simulink library "simCryogenics_lib"  (R2016a)
settings: Solver=VariableStepAuto  StartTime=0.0  StopTime=10.0  RelTol=1e-3
undefined symbols (not defined in the file or in its folder): gcbh, simscape
(part 3 of 4)

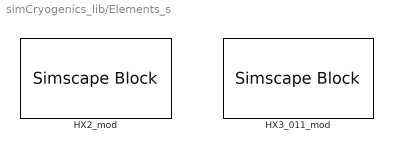
== system simCryogenics_lib/Elements_s ==
  HX2_mod : SimscapeBlock  DialogController=NetworkEngine.DynNeDlgSource  LoadFcn=simscape.compiler.sli.internal.callback('LoadFcn',gcbh);  SourceFile=simCryogenics.Elements_s.HeatEx2_mod  mask(HX2_mod){ComponentPath=simCryogenics.Elements_s.HeatEx2_mod, ComponentVariants=simCryogenics.Elements_s.HeatEx2_mod, ComponentVariantNames=HeatEx2_mod, ClassName=HeatEx2_mod, SchemaVersion=1, N=1, N_unit=1, N_conf=compiletime, Vh=2.3e-3, Vh_unit=m^3, Vh_conf=compiletime, Vc=2.3e-3, Vc_unit=m^3, Vc_conf=compiletime, M=13, M_unit=kg, M_conf=compiletime, Kh=0.6, Kh_unit=s*bar/kg, Kh_conf=compiletime, Kc=0.35, Kc_unit=s*bar/kg, Kc_conf=compiletime, Th0=10, Th0_unit=K, Th0_conf=compiletime, Ph0=16, Ph0_unit=bar, Ph0_conf=compiletime, Mh0=0.037, Mh0_unit=kg/s, Mh0_conf=compiletime, Tc0=4.5, Tc0_unit=K, Tc0_conf=compiletime, Pc0=1.1, Pc0_unit=bar, Pc0_conf=compiletime, Mc0=0.037, Mc0_unit=kg/s, Mc0_conf=compiletime, hhn=480, hhn_unit=J/s/K, hhn_conf=compiletime, hcn=480, hcn_unit=J/s/K, hcn_conf=compiletime, Mhn=1, Mhn_unit=kg/s, Mhn_conf=compiletime, Mcn=1, Mcn_unit=kg/s, Mcn_conf=compiletime, Thn=10, Thn_unit=K, Thn_conf=compiletime, Tcn=4.5, Tcn_unit=K, Tcn_conf=compiletime, Phn=16, Phn_unit=bar, Phn_conf=compiletime, Pcn=1.1, Pcn_unit=bar, Pcn_conf=compiletime, ex_mode=1, ex_mode_unit=1, ex_mode_conf=compiletime}
      mask prompts: N "Number of discrete elements"; Vh "First passage volume"; Vc "Sec. passage volume"; M "Heat exchanger mass"; Kh "First passage press. drop coeff."; Kc "Sec. passage press. drop coeff."; Th0 "Initial in1 temperature"; Ph0 "Initial in1 pressure"; Mh0 "Initial out1 flowrate"; Tc0 "Initial in2 temperature"; Pc0 "Initial out2 pressure"; Mc0 "Initial in2 flowrate"; hhn "Nominal exchange coefficient for hot pipe"; hcn "Nominal exchange coefficient for cold pipe"; Mhn "Nominal hot pipe flowrate"; Mcn "Nominal cold pipe flowrate"; Thn "Nominal hot pipe temperature"; Tcn "Nominal cold pipe temperature"; Phn "Nominal hot pipe pressure"; Pcn "Nominal cold pipe pressure"; ex_mode "Choice for h computation"
      mask help:
      | This component is a two branches cross-current heat Exchanger
      |
      | The following variables are imposed to others components: - in1 node : flow rate - out1 node : pressure and enthalpy - in2 node : enthalpy and flow rate - out2 node : pressure
      |
      | To ensure compilation, the heat Exchanger must be connected to components nodes that impose: - pressure and enthalpy on the in1 node - flowrate on the out1 node - flowrate and enthalpy on the in2 node - pressure on the out2 node
      |
      | Note : the initial temperature/flowrate/presure conditions should be equal to the actual value on the scheme (especially for heat exchangers connected to sources).
      |
      | All parameters must be positive
      mask init:
      | simscape.compiler.sli.internal.preinitmask(gcb);
      settings: CopyFcn=simscape.compiler.sli.internal.callback('CopyFcn',gcbh);  DeleteFcn=simscape.compiler.sli.internal.callback('DeleteFcn',gcbh);  ModelCloseFcn=simscape.compiler.sli.internal.callback('ModelCloseFcn',gcbh);  PreSaveFcn=simscape.compiler.sli.internal.callback('PreSaveFcn',gcbh);  PostSaveFcn=simscape.compiler.sli.internal.callback('PostSaveFcn',gcbh);  PreCopyFcn=simscape.compiler.sli.internal.callback('PreCopyFcn',gcbh);  PreDeleteFcn=simscape.compiler.sli.internal.callback('PreDeleteFcn',gcbh);
      mask Help: web(nesl_help(gcbh))
      mask TypeOptions N_conf: compiletime
      mask TypeOptions Vh_conf: compiletime
      mask TypeOptions Vc_conf: compiletime
      mask TypeOptions M_conf: compiletime
      mask TypeOptions Kh_conf: compiletime
      mask TypeOptions Kc_conf: compiletime
      mask TypeOptions Th0_conf: compiletime
      mask TypeOptions Ph0_conf: compiletime
      mask TypeOptions Mh0_conf: compiletime
      mask TypeOptions Tc0_conf: compiletime
      mask TypeOptions Pc0_conf: compiletime
      mask TypeOptions Mc0_conf: compiletime
      mask TypeOptions hhn_conf: compiletime
      mask TypeOptions hcn_conf: compiletime
      mask TypeOptions Mhn_conf: compiletime
      mask TypeOptions Mcn_conf: compiletime
      mask TypeOptions Thn_conf: compiletime
      mask TypeOptions Tcn_conf: compiletime
      mask TypeOptions Phn_conf: compiletime
      mask TypeOptions Pcn_conf: compiletime
      mask TypeOptions ex_mode_conf: compiletime | runtime
      mask Display:
      | disp('Simscape\n\n\n')
      | disp('\n\n\nHeatEx2_mod');
      | color('red');
      | port_label('RConn', 2,'out1');
      | port_label('RConn', 1,'in2');
      | port_label('LConn', 2,'in1');
      | port_label('LConn', 1,'out2');
  HX3_011_mod : SimscapeBlock  DialogController=NetworkEngine.DynNeDlgSource  LoadFcn=simscape.compiler.sli.internal.callback('LoadFcn',gcbh);  SourceFile=simCryogenics.Elements_s.HeatEx3_011_mod  mask(HX3_011_mod){ComponentPath=simCryogenics.Elements_s.HeatEx3_011_mod, ComponentVariants=simCryogenics.Elements_s.HeatEx3_011_mod, ComponentVariantNames=HeatEx3_011_mod, ClassName=HeatEx3_011_mod, SchemaVersion=1, N=8, N_unit=1, N_conf=compiletime, Vh=2.3e-3, Vh_unit=m^3, Vh_conf=compiletime, Vm=2.3e-3, Vm_unit=m^3, Vm_conf=compiletime, Vc=2.3e-3, Vc_unit=m^3, Vc_conf=compiletime, M=13, M_unit=kg, M_conf=compiletime, Kh=0, Kh_unit=s*bar/kg, Kh_conf=compiletime, Km=0, Km_unit=s*bar/kg, Km_conf=compiletime, Kc=0, Kc_unit=s*bar/kg, Kc_conf=compiletime, hn_h=400, hn_h_unit=W/K, hn_h_conf=compiletime, hn_m=400, hn_m_unit=W/K, hn_m_conf=compiletime, hn_c=400, hn_c_unit=W/K, hn_c_conf=compiletime, Th0=10, Th0_unit=K, Th0_conf=compiletime, Ph0=16, Ph0_unit=bar, Ph0_conf=compiletime, Mh0=0.037, Mh0_unit=kg/s, Mh0_conf=compiletime, Tm0=4.5, Tm0_unit=K, Tm0_conf=compiletime, Pm0=1.1, Pm0_unit=bar, Pm0_conf=compiletime, Mm0=0.037, Mm0_unit=kg/s, Mm0_conf=compiletime, Tc0=4.5, Tc0_unit=K, Tc0_conf=compiletime, Pc0=1.1, Pc0_unit=bar, Pc0_conf=compiletime, Mc0=0.037, Mc0_unit=kg/s, Mc0_conf=compiletime, Thn=10, Thn_unit=K, Thn_conf=compiletime, Phn=16, Phn_unit=bar, Phn_conf=compiletime, Mhn=0.037, Mhn_unit=kg/s, Mhn_conf=compiletime, Tmn=4.5, Tmn_unit=K, Tmn_conf=compiletime, Pmn=1.1, Pmn_unit=bar, Pmn_conf=compiletime, Mmn=0.037, Mmn_unit=kg/s, Mmn_conf=compiletime, Tcn=4.5, Tcn_unit=K, Tcn_conf=compiletime, Pcn=1.1, Pcn_unit=bar, Pcn_conf=compiletime, Mcn=0.037, Mcn_unit=kg/s, Mcn_conf=compiletime, ex_hp_bp=10, ex_hp_bp_unit=1, ex_hp_bp_conf=compiletime, ex_hp_mp=10, ex_hp_mp_unit=1, ex_hp_mp_conf=compiletime, ex_mp_bp=10, ex_mp_bp_unit=1, ex_mp_bp_conf=compiletime, ex_mode=1, ex_mode_unit=1, ex_mode_conf=compiletime, sensh=0, sensh_unit=1, sensh_conf=compiletime, sensm=1, sensm_unit=1, sensm_conf=compiletime, sensc=1, sensc_unit=1, sensc_conf=compiletime}
      mask prompts: N "Number of discrete elements"; Vh "First passage volume"; Vm "Second passage volume"; Vc "Third passage volume"; M "Heat exchanger mass"; Kh "First passage pressure drop"; Km "Second passage pressure drop"; Kc "Third passage pressure drop"; hn_h "Nominal ex. coef. for HP stream"; hn_m "Nominal ex. coef. for MP stream"; hn_c "Nominal ex. coef. for BP stream"; Th0 "Initial in1 temperature"; Ph0 "Initial in1 pressure"; Mh0 "Initial out1 flowrate"; Tm0 "Initial in2 temperature"; Pm0 "Initial out2 pressure"; Mm0 "Initial in2 flowrate"; Tc0 "Initial in3 temperature"; Pc0 "Initial out3 pressure"; Mc0 "Initial in3 flowrate"; Thn "Nominal in1 temperature"; Phn "Nominal in1 pressure"; Mhn "Nominal out1 flowrate"; Tmn "Nominal in2 temperature"; Pmn "Nominal out2 pressure"; Mmn "Nominal in2 flowrate"; Tcn "Nominal in3 temperature"; Pcn "Nominal out3 pressure"; Mcn "Nominal in3 flowrate"; ex_hp_bp "Number of interfaces between HP and BP streams"; ex_hp_mp "Number of interfaces between HP and MP streams"; ex_mp_bp "Number of interfaces between MP and BP streams"; ex_mode "Choice for h computation"; sensh "Sens hot flow"; sensm "Sens middle flow"; sensc "Sens cold flow"
      mask help:
      | This component is a three branches cross-current heat Exchanger
      |
      | The following variables are imposed to others components: - in1 node : pressure and enthalpy - out1 node :  flow rate - in2/3 node : enthalpy and flow rate - out2/3 node : pressure
      |
      | To ensure compilation, the heat Exchanger must be connected to components nodes that impose: - pressure and enthalpy on the in1 node - flowrate on the out1 node - flowrate and enthalpy on the in2/3 node - pressure on the out2/3 node
      |
      | Note : the initial temperature/flowrate/presure conditions should be equal to the actual value on the scheme (especially for heat exchangers connected to sources).
      |
      | All parameters must be positive
      mask init:
      | simscape.compiler.sli.internal.preinitmask(gcb);
      settings: CopyFcn=simscape.compiler.sli.internal.callback('CopyFcn',gcbh);  DeleteFcn=simscape.compiler.sli.internal.callback('DeleteFcn',gcbh);  ModelCloseFcn=simscape.compiler.sli.internal.callback('ModelCloseFcn',gcbh);  PreSaveFcn=simscape.compiler.sli.internal.callback('PreSaveFcn',gcbh);  PostSaveFcn=simscape.compiler.sli.internal.callback('PostSaveFcn',gcbh);  PreCopyFcn=simscape.compiler.sli.internal.callback('PreCopyFcn',gcbh);  PreDeleteFcn=simscape.compiler.sli.internal.callback('PreDeleteFcn',gcbh);
      mask Help: web(nesl_help(gcbh))
      mask TypeOptions N_conf: compiletime
      mask TypeOptions Vh_conf: compiletime
      mask TypeOptions Vm_conf: compiletime
      mask TypeOptions Vc_conf: compiletime
      mask TypeOptions M_conf: compiletime
      mask TypeOptions Kh_conf: compiletime
      mask TypeOptions Km_conf: compiletime
      mask TypeOptions Kc_conf: compiletime
      mask TypeOptions hn_h_conf: compiletime
      mask TypeOptions hn_m_conf: compiletime
      mask TypeOptions hn_c_conf: compiletime
      mask TypeOptions Th0_conf: compiletime
      mask TypeOptions Ph0_conf: compiletime
      mask TypeOptions Mh0_conf: compiletime
      mask TypeOptions Tm0_conf: compiletime
      mask TypeOptions Pm0_conf: compiletime
      mask TypeOptions Mm0_conf: compiletime
      mask TypeOptions Tc0_conf: compiletime
      mask TypeOptions Pc0_conf: compiletime
      mask TypeOptions Mc0_conf: compiletime
      mask TypeOptions Thn_conf: compiletime
      mask TypeOptions Phn_conf: compiletime
      mask TypeOptions Mhn_conf: compiletime
      mask TypeOptions Tmn_conf: compiletime
      mask TypeOptions Pmn_conf: compiletime
      mask TypeOptions Mmn_conf: compiletime
      mask TypeOptions Tcn_conf: compiletime
      mask TypeOptions Pcn_conf: compiletime
      mask TypeOptions Mcn_conf: compiletime
      mask TypeOptions ex_hp_bp_conf: compiletime
      mask TypeOptions ex_hp_mp_conf: compiletime
      mask TypeOptions ex_mp_bp_conf: compiletime
      mask TypeOptions ex_mode_conf: compiletime | runtime
      mask TypeOptions sensh_conf: compiletime
      mask TypeOptions sensm_conf: compiletime
      mask TypeOptions sensc_conf: compiletime
      mask Display:
      | disp('Simscape\n\n\n')
      | disp('\n\n\nHeatEx3_011_mod');
      | color('red');
      | port_label('LConn', 3,'in1');
      | port_label('LConn', 2,'out2');
      | port_label('LConn', 1,'out3');
      | port_label('RConn', 3,'out1');
      | port_label('RConn', 2,'in2');
      | port_label('RConn', 1,'in3');

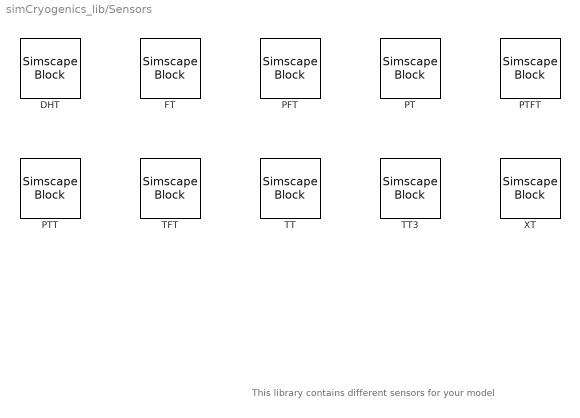
== system simCryogenics_lib/Sensors ==
  note: This library contains different sensors for your model
  DHT : SimscapeBlock  DialogController=NetworkEngine.DynNeDlgSource  LoadFcn=simscape.compiler.sli.internal.callback('LoadFcn',gcbh);  SourceFile=simCryogenics.Sensors.DHT  mask(DHT){ComponentPath=simCryogenics.Sensors.DHT, ComponentVariants=simCryogenics.Sensors.DHT, ComponentVariantNames=DHT, ClassName=DHT, SchemaVersion=1}
      mask init:
      | simscape.compiler.sli.internal.preinitmask(gcb);
      settings: CopyFcn=simscape.compiler.sli.internal.callback('CopyFcn',gcbh);  DeleteFcn=simscape.compiler.sli.internal.callback('DeleteFcn',gcbh);  ModelCloseFcn=simscape.compiler.sli.internal.callback('ModelCloseFcn',gcbh);  PreSaveFcn=simscape.compiler.sli.internal.callback('PreSaveFcn',gcbh);  PostSaveFcn=simscape.compiler.sli.internal.callback('PostSaveFcn',gcbh);  PreCopyFcn=simscape.compiler.sli.internal.callback('PreCopyFcn',gcbh);  PreDeleteFcn=simscape.compiler.sli.internal.callback('PreDeleteFcn',gcbh);
      mask Help: web(nesl_help(gcbh))
      mask Display:
      | color('red');
      | port_label('RConn', 1,'');
      | port_label('LConn', 2,'');
      | port_label('LConn', 1,'');
  FT : SimscapeBlock  DialogController=NetworkEngine.DynNeDlgSource  LoadFcn=simscape.compiler.sli.internal.callback('LoadFcn',gcbh);  SourceFile=simCryogenics.Sensors.FT  mask(FT){ComponentPath=simCryogenics.Sensors.FT, ComponentVariants=simCryogenics.Sensors.FT, ComponentVariantNames=FT, ClassName=FT, SchemaVersion=1}
      mask help: This component is a perfect flow sensor
      mask init:
      | simscape.compiler.sli.internal.preinitmask(gcb);
      settings: CopyFcn=simscape.compiler.sli.internal.callback('CopyFcn',gcbh);  DeleteFcn=simscape.compiler.sli.internal.callback('DeleteFcn',gcbh);  ModelCloseFcn=simscape.compiler.sli.internal.callback('ModelCloseFcn',gcbh);  PreSaveFcn=simscape.compiler.sli.internal.callback('PreSaveFcn',gcbh);  PostSaveFcn=simscape.compiler.sli.internal.callback('PostSaveFcn',gcbh);  PreCopyFcn=simscape.compiler.sli.internal.callback('PreCopyFcn',gcbh);  PreDeleteFcn=simscape.compiler.sli.internal.callback('PreDeleteFcn',gcbh);
      mask Help: web(nesl_help(gcbh))
      mask Display:
      | color('red');
      | port_label('RConn', 1,'');
      | port_label('LConn', 1,'');
  PFT : SimscapeBlock  DialogController=NetworkEngine.DynNeDlgSource  LoadFcn=simscape.compiler.sli.internal.callback('LoadFcn',gcbh);  SourceFile=simCryogenics.Sensors.PFT  mask(PFT){ComponentPath=simCryogenics.Sensors.PFT, ComponentVariants=simCryogenics.Sensors.PFT, ComponentVariantNames=PFT, ClassName=PFT, SchemaVersion=1}
      mask help: This component is a perfect pressure and temperature sensor
      mask init:
      | simscape.compiler.sli.internal.preinitmask(gcb);
      settings: CopyFcn=simscape.compiler.sli.internal.callback('CopyFcn',gcbh);  DeleteFcn=simscape.compiler.sli.internal.callback('DeleteFcn',gcbh);  ModelCloseFcn=simscape.compiler.sli.internal.callback('ModelCloseFcn',gcbh);  PreSaveFcn=simscape.compiler.sli.internal.callback('PreSaveFcn',gcbh);  PostSaveFcn=simscape.compiler.sli.internal.callback('PostSaveFcn',gcbh);  PreCopyFcn=simscape.compiler.sli.internal.callback('PreCopyFcn',gcbh);  PreDeleteFcn=simscape.compiler.sli.internal.callback('PreDeleteFcn',gcbh);
      mask Help: web(nesl_help(gcbh))
      mask Display:
      | color('red');
      | port_label('RConn', 2,'F');
      | port_label('RConn', 1,'P');
      | port_label('LConn', 1,'');
  PT : SimscapeBlock  DialogController=NetworkEngine.DynNeDlgSource  LoadFcn=simscape.compiler.sli.internal.callback('LoadFcn',gcbh);  SourceFile=simCryogenics.Sensors.PT  mask(PT){ComponentPath=simCryogenics.Sensors.PT, ComponentVariants=simCryogenics.Sensors.PT, ComponentVariantNames=PT, ClassName=PT, SchemaVersion=1}
      mask help: This component is a perfect pressure sensor
      mask init:
      | simscape.compiler.sli.internal.preinitmask(gcb);
      settings: CopyFcn=simscape.compiler.sli.internal.callback('CopyFcn',gcbh);  DeleteFcn=simscape.compiler.sli.internal.callback('DeleteFcn',gcbh);  ModelCloseFcn=simscape.compiler.sli.internal.callback('ModelCloseFcn',gcbh);  PreSaveFcn=simscape.compiler.sli.internal.callback('PreSaveFcn',gcbh);  PostSaveFcn=simscape.compiler.sli.internal.callback('PostSaveFcn',gcbh);  PreCopyFcn=simscape.compiler.sli.internal.callback('PreCopyFcn',gcbh);  PreDeleteFcn=simscape.compiler.sli.internal.callback('PreDeleteFcn',gcbh);
      mask Help: web(nesl_help(gcbh))
      mask Display:
      | color('red');
      | port_label('RConn', 1,'');
      | port_label('LConn', 1,'');
  PTFT : SimscapeBlock  DialogController=NetworkEngine.DynNeDlgSource  LoadFcn=simscape.compiler.sli.internal.callback('LoadFcn',gcbh);  SourceFile=simCryogenics.Sensors.PTFT  mask(PTFT){ComponentPath=simCryogenics.Sensors.PTFT, ComponentVariants=simCryogenics.Sensors.PTFT, ComponentVariantNames=PTFT, ClassName=PTFT, SchemaVersion=1}
      mask help: This component is a perfect pressure and temperature sensor
      mask init:
      | simscape.compiler.sli.internal.preinitmask(gcb);
      settings: CopyFcn=simscape.compiler.sli.internal.callback('CopyFcn',gcbh);  DeleteFcn=simscape.compiler.sli.internal.callback('DeleteFcn',gcbh);  ModelCloseFcn=simscape.compiler.sli.internal.callback('ModelCloseFcn',gcbh);  PreSaveFcn=simscape.compiler.sli.internal.callback('PreSaveFcn',gcbh);  PostSaveFcn=simscape.compiler.sli.internal.callback('PostSaveFcn',gcbh);  PreCopyFcn=simscape.compiler.sli.internal.callback('PreCopyFcn',gcbh);  PreDeleteFcn=simscape.compiler.sli.internal.callback('PreDeleteFcn',gcbh);
      mask Help: web(nesl_help(gcbh))
      mask Display:
      | color('red');
      | port_label('RConn', 3,'F');
      | port_label('RConn', 2,'T');
      | port_label('RConn', 1,'P');
      | port_label('LConn', 1,'');
  PTT : SimscapeBlock  DialogController=NetworkEngine.DynNeDlgSource  LoadFcn=simscape.compiler.sli.internal.callback('LoadFcn',gcbh);  SourceFile=simCryogenics.Sensors.PTT  mask(PTT){ComponentPath=simCryogenics.Sensors.PTT, ComponentVariants=simCryogenics.Sensors.PTT, ComponentVariantNames=PTT, ClassName=PTT, SchemaVersion=1}
      mask help: This component is a perfect pressure and temperature sensor
      mask init:
      | simscape.compiler.sli.internal.preinitmask(gcb);
      settings: CopyFcn=simscape.compiler.sli.internal.callback('CopyFcn',gcbh);  DeleteFcn=simscape.compiler.sli.internal.callback('DeleteFcn',gcbh);  ModelCloseFcn=simscape.compiler.sli.internal.callback('ModelCloseFcn',gcbh);  PreSaveFcn=simscape.compiler.sli.internal.callback('PreSaveFcn',gcbh);  PostSaveFcn=simscape.compiler.sli.internal.callback('PostSaveFcn',gcbh);  PreCopyFcn=simscape.compiler.sli.internal.callback('PreCopyFcn',gcbh);  PreDeleteFcn=simscape.compiler.sli.internal.callback('PreDeleteFcn',gcbh);
      mask Help: web(nesl_help(gcbh))
      mask Display:
      | color('red');
      | port_label('RConn', 2,'T');
      | port_label('RConn', 1,'P');
      | port_label('LConn', 1,'');
  TFT : SimscapeBlock  DialogController=NetworkEngine.DynNeDlgSource  LoadFcn=simscape.compiler.sli.internal.callback('LoadFcn',gcbh);  SourceFile=simCryogenics.Sensors.TFT  mask(TFT){ComponentPath=simCryogenics.Sensors.TFT, ComponentVariants=simCryogenics.Sensors.TFT, ComponentVariantNames=TFT, ClassName=TFT, SchemaVersion=1}
      mask help: This component is a perfect pressure and temperature sensor
      mask init:
      | simscape.compiler.sli.internal.preinitmask(gcb);
      settings: CopyFcn=simscape.compiler.sli.internal.callback('CopyFcn',gcbh);  DeleteFcn=simscape.compiler.sli.internal.callback('DeleteFcn',gcbh);  ModelCloseFcn=simscape.compiler.sli.internal.callback('ModelCloseFcn',gcbh);  PreSaveFcn=simscape.compiler.sli.internal.callback('PreSaveFcn',gcbh);  PostSaveFcn=simscape.compiler.sli.internal.callback('PostSaveFcn',gcbh);  PreCopyFcn=simscape.compiler.sli.internal.callback('PreCopyFcn',gcbh);  PreDeleteFcn=simscape.compiler.sli.internal.callback('PreDeleteFcn',gcbh);
      mask Help: web(nesl_help(gcbh))
      mask Display:
      | color('red');
      | port_label('RConn', 2,'F');
      | port_label('RConn', 1,'T');
      | port_label('LConn', 1,'');
  TT : SimscapeBlock  DialogController=NetworkEngine.DynNeDlgSource  LoadFcn=simscape.compiler.sli.internal.callback('LoadFcn',gcbh);  SourceFile=simCryogenics.Sensors.TT  mask(TT){ComponentPath=simCryogenics.Sensors.TT, ComponentVariants=simCryogenics.Sensors.TT, ComponentVariantNames=TT, ClassName=TT, SchemaVersion=1}
      mask help: This component is a perfect temperature sensor
      mask init:
      | simscape.compiler.sli.internal.preinitmask(gcb);
      settings: CopyFcn=simscape.compiler.sli.internal.callback('CopyFcn',gcbh);  DeleteFcn=simscape.compiler.sli.internal.callback('DeleteFcn',gcbh);  ModelCloseFcn=simscape.compiler.sli.internal.callback('ModelCloseFcn',gcbh);  PreSaveFcn=simscape.compiler.sli.internal.callback('PreSaveFcn',gcbh);  PostSaveFcn=simscape.compiler.sli.internal.callback('PostSaveFcn',gcbh);  PreCopyFcn=simscape.compiler.sli.internal.callback('PreCopyFcn',gcbh);  PreDeleteFcn=simscape.compiler.sli.internal.callback('PreDeleteFcn',gcbh);
      mask Help: web(nesl_help(gcbh))
      mask Display:
      | color('red');
      | port_label('RConn', 1,'');
      | port_label('LConn', 1,'');
  TT3 : SimscapeBlock  DialogController=NetworkEngine.DynNeDlgSource  LoadFcn=simscape.compiler.sli.internal.callback('LoadFcn',gcbh);  SourceFile=simCryogenics.Sensors.TT3  mask(TT3){ComponentPath=simCryogenics.Sensors.TT3, ComponentVariants=simCryogenics.Sensors.TT3, ComponentVariantNames=TT3, ClassName=TT3, SchemaVersion=1}
      mask help: This component is a perfect pressure and temperature sensor
      mask init:
      | simscape.compiler.sli.internal.preinitmask(gcb);
      settings: CopyFcn=simscape.compiler.sli.internal.callback('CopyFcn',gcbh);  DeleteFcn=simscape.compiler.sli.internal.callback('DeleteFcn',gcbh);  ModelCloseFcn=simscape.compiler.sli.internal.callback('ModelCloseFcn',gcbh);  PreSaveFcn=simscape.compiler.sli.internal.callback('PreSaveFcn',gcbh);  PostSaveFcn=simscape.compiler.sli.internal.callback('PostSaveFcn',gcbh);  PreCopyFcn=simscape.compiler.sli.internal.callback('PreCopyFcn',gcbh);  PreDeleteFcn=simscape.compiler.sli.internal.callback('PreDeleteFcn',gcbh);
      mask Help: web(nesl_help(gcbh))
      mask Display:
      | color('red');
      | port_label('RConn', 1,'T');
      | port_label('LConn', 3,'');
      | port_label('LConn', 2,'');
      | port_label('LConn', 1,'');
  XT : SimscapeBlock  DialogController=NetworkEngine.DynNeDlgSource  LoadFcn=simscape.compiler.sli.internal.callback('LoadFcn',gcbh);  SourceFile=simCryogenics.Sensors.XT  mask(XT){ComponentPath=simCryogenics.Sensors.XT, ComponentVariants=simCryogenics.Sensors.XT, ComponentVariantNames=XT, ClassName=XT, SchemaVersion=1}
      mask help: This component is a perfect quality sensor
      mask init:
      | simscape.compiler.sli.internal.preinitmask(gcb);
      settings: CopyFcn=simscape.compiler.sli.internal.callback('CopyFcn',gcbh);  DeleteFcn=simscape.compiler.sli.internal.callback('DeleteFcn',gcbh);  ModelCloseFcn=simscape.compiler.sli.internal.callback('ModelCloseFcn',gcbh);  PreSaveFcn=simscape.compiler.sli.internal.callback('PreSaveFcn',gcbh);  PostSaveFcn=simscape.compiler.sli.internal.callback('PostSaveFcn',gcbh);  PreCopyFcn=simscape.compiler.sli.internal.callback('PreCopyFcn',gcbh);  PreDeleteFcn=simscape.compiler.sli.internal.callback('PreDeleteFcn',gcbh);
      mask Help: web(nesl_help(gcbh))
      mask Display:
      | color('red');
      | port_label('RConn', 1,'');
      | port_label('LConn', 1,'');

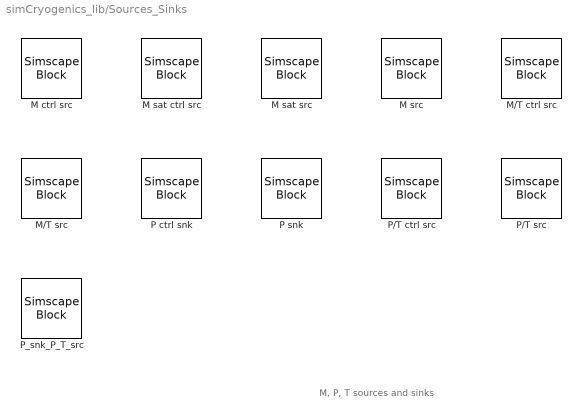
== system simCryogenics_lib/Sources_Sinks ==
  note: M, P, T sources and sinks
  M ctrl src : SimscapeBlock  DialogController=NetworkEngine.DynNeDlgSource  LoadFcn=simscape.compiler.sli.internal.callback('LoadFcn',gcbh);  SourceFile=simCryogenics.Sources_Sinks.M_ctrl_src  mask(M ctrl src){ComponentPath=simCryogenics.Sources_Sinks.M_ctrl_src, ComponentVariants=simCryogenics.Sources_Sinks.M_ctrl_src, ComponentVariantNames=M_ctrl_src, ClassName=M_ctrl_src, SchemaVersion=1}
      mask help: This block is a perfect mass flow rate source. It's imposed a constant mass flow regardless of the pressure and temperature. The control input of this component define the value of the mass flow, the unit of the mass flow is [kg/s]
      mask init:
      | simscape.compiler.sli.internal.preinitmask(gcb);
      settings: CopyFcn=simscape.compiler.sli.internal.callback('CopyFcn',gcbh);  DeleteFcn=simscape.compiler.sli.internal.callback('DeleteFcn',gcbh);  ModelCloseFcn=simscape.compiler.sli.internal.callback('ModelCloseFcn',gcbh);  PreSaveFcn=simscape.compiler.sli.internal.callback('PreSaveFcn',gcbh);  PostSaveFcn=simscape.compiler.sli.internal.callback('PostSaveFcn',gcbh);  PreCopyFcn=simscape.compiler.sli.internal.callback('PreCopyFcn',gcbh);  PreDeleteFcn=simscape.compiler.sli.internal.callback('PreDeleteFcn',gcbh);
      mask Help: web(nesl_help(gcbh))
      mask Display:
      | color('red');
      | port_label('RConn', 1,'');
      | port_label('LConn', 1,'');
  M sat ctrl src : SimscapeBlock  DialogController=NetworkEngine.DynNeDlgSource  LoadFcn=simscape.compiler.sli.internal.callback('LoadFcn',gcbh);  SourceFile=simCryogenics.Sources_Sinks.M_sat_ctrl_src  mask(M sat ctrl src){ComponentPath=simCryogenics.Sources_Sinks.M_sat_ctrl_src, ComponentVariants=simCryogenics.Sources_Sinks.M_sat_ctrl_src, ComponentVariantNames=M_sat_ctrl_src, ClassName=M_sat_ctrl_src, SchemaVersion=1}
      mask help:
      | This block is a perfect satured mass flow rate source. It impose a saturated mass flow regardless the pressure.
      |
      | Input flowrate F must be greather than zero Input mixture quality X must be comprise beetween 0 and 1
      mask init:
      | simscape.compiler.sli.internal.preinitmask(gcb);
      settings: CopyFcn=simscape.compiler.sli.internal.callback('CopyFcn',gcbh);  DeleteFcn=simscape.compiler.sli.internal.callback('DeleteFcn',gcbh);  ModelCloseFcn=simscape.compiler.sli.internal.callback('ModelCloseFcn',gcbh);  PreSaveFcn=simscape.compiler.sli.internal.callback('PreSaveFcn',gcbh);  PostSaveFcn=simscape.compiler.sli.internal.callback('PostSaveFcn',gcbh);  PreCopyFcn=simscape.compiler.sli.internal.callback('PreCopyFcn',gcbh);  PreDeleteFcn=simscape.compiler.sli.internal.callback('PreDeleteFcn',gcbh);
      mask Help: web(nesl_help(gcbh))
      mask Display:
      | color('red');
      | port_label('RConn', 1,'');
      | port_label('LConn', 2,'X');
      | port_label('LConn', 1,'F');
  M sat src : SimscapeBlock  DialogController=NetworkEngine.DynNeDlgSource  LoadFcn=simscape.compiler.sli.internal.callback('LoadFcn',gcbh);  SourceFile=simCryogenics.Sources_Sinks.M_sat_src  mask(M sat src){ComponentPath=simCryogenics.Sources_Sinks.M_sat_src, ComponentVariants=simCryogenics.Sources_Sinks.M_sat_src, ComponentVariantNames=M_sat_src, ClassName=M_sat_src, SchemaVersion=1, M=0.01, M_unit=kg/s, M_conf=compiletime, Xmix=0.5, Xmix_unit=1, Xmix_conf=compiletime}
      mask prompts: M "Flowrate"; Xmix "Mixture Quality"
      mask help:
      | This block is a perfect satured mass flow rate source. It impose a constant saturated mass flow regardless the pressure.
      |
      | Flowrate must be greather than zero Mixture quality must be comprise beetween 0 and 1
      mask init:
      | simscape.compiler.sli.internal.preinitmask(gcb);
      settings: CopyFcn=simscape.compiler.sli.internal.callback('CopyFcn',gcbh);  DeleteFcn=simscape.compiler.sli.internal.callback('DeleteFcn',gcbh);  ModelCloseFcn=simscape.compiler.sli.internal.callback('ModelCloseFcn',gcbh);  PreSaveFcn=simscape.compiler.sli.internal.callback('PreSaveFcn',gcbh);  PostSaveFcn=simscape.compiler.sli.internal.callback('PostSaveFcn',gcbh);  PreCopyFcn=simscape.compiler.sli.internal.callback('PreCopyFcn',gcbh);  PreDeleteFcn=simscape.compiler.sli.internal.callback('PreDeleteFcn',gcbh);
      mask Help: web(nesl_help(gcbh))
      mask TypeOptions M_conf: compiletime
      mask TypeOptions Xmix_conf: compiletime
      mask Display:
      | color('red');
      | port_label('RConn', 1,'');
  M src : SimscapeBlock  DialogController=NetworkEngine.DynNeDlgSource  LoadFcn=simscape.compiler.sli.internal.callback('LoadFcn',gcbh);  SourceFile=simCryogenics.Sources_Sinks.M_src  mask(M src){ComponentPath=simCryogenics.Sources_Sinks.M_src, ComponentVariants=simCryogenics.Sources_Sinks.M_src, ComponentVariantNames=M_src, ClassName=M_src, SchemaVersion=1, M=0.01, M_unit=kg/s, M_conf=compiletime}
      mask prompts: M "Flowrate"
      mask help: This block is a perfect mass flow rate source. It's imposed a constant mass flow regardless of the pressure and temperature. The parameter of this component define the value of the mass flow, the unit of the mass flow is [kg/s].
      mask init:
      | simscape.compiler.sli.internal.preinitmask(gcb);
      settings: CopyFcn=simscape.compiler.sli.internal.callback('CopyFcn',gcbh);  DeleteFcn=simscape.compiler.sli.internal.callback('DeleteFcn',gcbh);  ModelCloseFcn=simscape.compiler.sli.internal.callback('ModelCloseFcn',gcbh);  PreSaveFcn=simscape.compiler.sli.internal.callback('PreSaveFcn',gcbh);  PostSaveFcn=simscape.compiler.sli.internal.callback('PostSaveFcn',gcbh);  PreCopyFcn=simscape.compiler.sli.internal.callback('PreCopyFcn',gcbh);  PreDeleteFcn=simscape.compiler.sli.internal.callback('PreDeleteFcn',gcbh);
      mask Help: web(nesl_help(gcbh))
      mask TypeOptions M_conf: compiletime | runtime
      mask Display:
      | color('red');
      | port_label('RConn', 1,'');
  M/T ctrl src : SimscapeBlock  DialogController=NetworkEngine.DynNeDlgSource  LoadFcn=simscape.compiler.sli.internal.callback('LoadFcn',gcbh);  SourceFile=simCryogenics.Sources_Sinks.M_T_ctrl_src  mask(M/T ctrl src){ComponentPath=simCryogenics.Sources_Sinks.M_T_ctrl_src, ComponentVariants=simCryogenics.Sources_Sinks.M_T_ctrl_src, ComponentVariantNames=M_T_ctrl_src, ClassName=M_T_ctrl_src, SchemaVersion=1}
      mask help: This block is a perfect mass flow rate and temperature source. It's imposed a constant mass flow and temperature regardless of the pressure. The first input of this component define the value of the mass flow, the unit of the mass flow is [kg/s]. The second input of this compoent define the value of the temperature, the unit of the temperature is [K].
      mask init:
      | simscape.compiler.sli.internal.preinitmask(gcb);
      settings: CopyFcn=simscape.compiler.sli.internal.callback('CopyFcn',gcbh);  DeleteFcn=simscape.compiler.sli.internal.callback('DeleteFcn',gcbh);  ModelCloseFcn=simscape.compiler.sli.internal.callback('ModelCloseFcn',gcbh);  PreSaveFcn=simscape.compiler.sli.internal.callback('PreSaveFcn',gcbh);  PostSaveFcn=simscape.compiler.sli.internal.callback('PostSaveFcn',gcbh);  PreCopyFcn=simscape.compiler.sli.internal.callback('PreCopyFcn',gcbh);  PreDeleteFcn=simscape.compiler.sli.internal.callback('PreDeleteFcn',gcbh);
      mask Help: web(nesl_help(gcbh))
      mask Display:
      | color('red');
      | port_label('RConn', 1,'');
      | port_label('LConn', 2,'T');
      | port_label('LConn', 1,'M');
  M/T src : SimscapeBlock  DialogController=NetworkEngine.DynNeDlgSource  LoadFcn=simscape.compiler.sli.internal.callback('LoadFcn',gcbh);  SourceFile=simCryogenics.Sources_Sinks.M_T_src  mask(M/T src){ComponentPath=simCryogenics.Sources_Sinks.M_T_src, ComponentVariants=simCryogenics.Sources_Sinks.M_T_src, ComponentVariantNames=M_T_src, ClassName=M_T_src, SchemaVersion=1, M=0.01, M_unit=kg/s, M_conf=compiletime, T=300, T_unit=K, T_conf=compiletime}
      mask prompts: M "Mass flow rate [kg/s]"; T "Température [K]"
      mask help: This block is a perfect mass flow rate and temperature source. It's imposed a constant mass flow and temperature regardless of the pressure. The first parameter of this component define the value of the mass flow, the unit of the mass flow is [kg/s]. The second parameter of this compoent define the value of the temperature, the unit of the temperature is [K].
      mask init:
      | simscape.compiler.sli.internal.preinitmask(gcb);
      settings: CopyFcn=simscape.compiler.sli.internal.callback('CopyFcn',gcbh);  DeleteFcn=simscape.compiler.sli.internal.callback('DeleteFcn',gcbh);  ModelCloseFcn=simscape.compiler.sli.internal.callback('ModelCloseFcn',gcbh);  PreSaveFcn=simscape.compiler.sli.internal.callback('PreSaveFcn',gcbh);  PostSaveFcn=simscape.compiler.sli.internal.callback('PostSaveFcn',gcbh);  PreCopyFcn=simscape.compiler.sli.internal.callback('PreCopyFcn',gcbh);  PreDeleteFcn=simscape.compiler.sli.internal.callback('PreDeleteFcn',gcbh);
      mask Help: web(nesl_help(gcbh))
      mask TypeOptions M_conf: compiletime | runtime
      mask TypeOptions T_conf: compiletime | runtime
      mask Display:
      | color('red');
      | port_label('RConn', 1,'');
  P ctrl snk : SimscapeBlock  DialogController=NetworkEngine.DynNeDlgSource  LoadFcn=simscape.compiler.sli.internal.callback('LoadFcn',gcbh);  SourceFile=simCryogenics.Sources_Sinks.P_ctrl_snk  mask(P ctrl snk){ComponentPath=simCryogenics.Sources_Sinks.P_ctrl_snk, ComponentVariants=simCryogenics.Sources_Sinks.P_ctrl_snk, ComponentVariantNames=P_ctrl_snk, ClassName=P_ctrl_snk, SchemaVersion=1}
      mask help: This block is a perfect pressure sink. It's imposed a constant pressure regardless of the mass flow and the temperature. The ipnut of this component define the value of the pressure, the unit of the pressure is [kg/s].
      mask init:
      | simscape.compiler.sli.internal.preinitmask(gcb);
      settings: CopyFcn=simscape.compiler.sli.internal.callback('CopyFcn',gcbh);  DeleteFcn=simscape.compiler.sli.internal.callback('DeleteFcn',gcbh);  ModelCloseFcn=simscape.compiler.sli.internal.callback('ModelCloseFcn',gcbh);  PreSaveFcn=simscape.compiler.sli.internal.callback('PreSaveFcn',gcbh);  PostSaveFcn=simscape.compiler.sli.internal.callback('PostSaveFcn',gcbh);  PreCopyFcn=simscape.compiler.sli.internal.callback('PreCopyFcn',gcbh);  PreDeleteFcn=simscape.compiler.sli.internal.callback('PreDeleteFcn',gcbh);
      mask Help: web(nesl_help(gcbh))
      mask Display:
      | color('red');
      | port_label('RConn', 1,'');
      | port_label('LConn', 1,'');
  P snk : SimscapeBlock  DialogController=NetworkEngine.DynNeDlgSource  LoadFcn=simscape.compiler.sli.internal.callback('LoadFcn',gcbh);  SourceFile=simCryogenics.Sources_Sinks.P_snk  mask(P snk){ComponentPath=simCryogenics.Sources_Sinks.P_snk, ComponentVariants=simCryogenics.Sources_Sinks.P_snk, ComponentVariantNames=P_snk, ClassName=P_snk, SchemaVersion=1, P=0, P_unit=bar, P_conf=compiletime}
      mask prompts: P "Pressure"
      mask help: This block is a perfect pressure sink. It's imposed a constant pressure regardless of the mass flow and the temperature. The parameter of this component define the value of the pressure, the unit of the pressure is [bar].
      mask init:
      | simscape.compiler.sli.internal.preinitmask(gcb);
      settings: CopyFcn=simscape.compiler.sli.internal.callback('CopyFcn',gcbh);  DeleteFcn=simscape.compiler.sli.internal.callback('DeleteFcn',gcbh);  ModelCloseFcn=simscape.compiler.sli.internal.callback('ModelCloseFcn',gcbh);  PreSaveFcn=simscape.compiler.sli.internal.callback('PreSaveFcn',gcbh);  PostSaveFcn=simscape.compiler.sli.internal.callback('PostSaveFcn',gcbh);  PreCopyFcn=simscape.compiler.sli.internal.callback('PreCopyFcn',gcbh);  PreDeleteFcn=simscape.compiler.sli.internal.callback('PreDeleteFcn',gcbh);
      mask Help: web(nesl_help(gcbh))
      mask TypeOptions P_conf: compiletime | runtime
      mask Display:
      | color('red');
      | port_label('RConn', 1,'');
  P/T ctrl src : SimscapeBlock  DialogController=NetworkEngine.DynNeDlgSource  LoadFcn=simscape.compiler.sli.internal.callback('LoadFcn',gcbh);  SourceFile=simCryogenics.Sources_Sinks.P_T_ctrl_src  mask(P/T ctrl src){ComponentPath=simCryogenics.Sources_Sinks.P_T_ctrl_src, ComponentVariants=simCryogenics.Sources_Sinks.P_T_ctrl_src, ComponentVariantNames=P_T_ctrl_src, ClassName=P_T_ctrl_src, SchemaVersion=1}
      mask help: This block is a perfect pressure and temperature source. It's imposed a constant pressure and temperature regardless of the mass flow. The first input of this component define the value of the pressure, the unit of the mass flow is [bar]. The second input of this compoent define the value of the temperature, the unit of the temperature is [K].
      mask init:
      | simscape.compiler.sli.internal.preinitmask(gcb);
      settings: CopyFcn=simscape.compiler.sli.internal.callback('CopyFcn',gcbh);  DeleteFcn=simscape.compiler.sli.internal.callback('DeleteFcn',gcbh);  ModelCloseFcn=simscape.compiler.sli.internal.callback('ModelCloseFcn',gcbh);  PreSaveFcn=simscape.compiler.sli.internal.callback('PreSaveFcn',gcbh);  PostSaveFcn=simscape.compiler.sli.internal.callback('PostSaveFcn',gcbh);  PreCopyFcn=simscape.compiler.sli.internal.callback('PreCopyFcn',gcbh);  PreDeleteFcn=simscape.compiler.sli.internal.callback('PreDeleteFcn',gcbh);
      mask Help: web(nesl_help(gcbh))
      mask Display:
      | color('red');
      | port_label('RConn', 1,'');
      | port_label('LConn', 2,'T');
      | port_label('LConn', 1,'P');
  P/T src : SimscapeBlock  DialogController=NetworkEngine.DynNeDlgSource  LoadFcn=simscape.compiler.sli.internal.callback('LoadFcn',gcbh);  SourceFile=simCryogenics.Sources_Sinks.P_T_src  mask(P/T src){ComponentPath=simCryogenics.Sources_Sinks.P_T_src, ComponentVariants=simCryogenics.Sources_Sinks.P_T_src, ComponentVariantNames=P_T_src, ClassName=P_T_src, SchemaVersion=1, P=1, P_unit=bar, P_conf=compiletime, T=300, T_unit=K, T_conf=compiletime}
      mask prompts: P "Pressure [bar]"; T "Temperature [K]"
      mask help: This block is a perfect pressure and temperature source. It's imposed a constant pressure and temperature regardless of the mass flow. The first argument of this component define the value of the pressure, the unit of the mass flow is [bar]. The second argument of this compoent define the value of the temperature, the unit of the temperature is [K].
      mask init:
      | simscape.compiler.sli.internal.preinitmask(gcb);
      settings: CopyFcn=simscape.compiler.sli.internal.callback('CopyFcn',gcbh);  DeleteFcn=simscape.compiler.sli.internal.callback('DeleteFcn',gcbh);  ModelCloseFcn=simscape.compiler.sli.internal.callback('ModelCloseFcn',gcbh);  PreSaveFcn=simscape.compiler.sli.internal.callback('PreSaveFcn',gcbh);  PostSaveFcn=simscape.compiler.sli.internal.callback('PostSaveFcn',gcbh);  PreCopyFcn=simscape.compiler.sli.internal.callback('PreCopyFcn',gcbh);  PreDeleteFcn=simscape.compiler.sli.internal.callback('PreDeleteFcn',gcbh);
      mask Help: web(nesl_help(gcbh))
      mask TypeOptions P_conf: compiletime | runtime
      mask TypeOptions T_conf: compiletime | runtime
      mask Display:
      | color('red');
      | port_label('RConn', 1,'');
  P_snk_P_T_src : SimscapeBlock  DialogController=NetworkEngine.DynNeDlgSource  LoadFcn=simscape.compiler.sli.internal.callback('LoadFcn',gcbh);  SourceFile=simCryogenics.Sources_Sinks.P_snk_P_T_src  mask(P_snk_P_T_src){ComponentPath=simCryogenics.Sources_Sinks.P_snk_P_T_src, ComponentVariants=simCryogenics.Sources_Sinks.P_snk_P_T_src, ComponentVariantNames=P_snk_P_T_src, ClassName=P_snk_P_T_src, SchemaVersion=1, P=5, P_unit=bar, P_conf=compiletime}
      mask prompts: P "Pressure [bar]"
      mask help: This block is a perfect pressure and temperature source. It's imposed a constant pressure and temperature regardless of the mass flow. The first argument of this component define the value of the pressure, the unit of the mass flow is [bar]. The second argument of this compoent define the value of the temperature, the unit of the temperature is [K].
      mask init:
      | simscape.compiler.sli.internal.preinitmask(gcb);
      settings: CopyFcn=simscape.compiler.sli.internal.callback('CopyFcn',gcbh);  DeleteFcn=simscape.compiler.sli.internal.callback('DeleteFcn',gcbh);  ModelCloseFcn=simscape.compiler.sli.internal.callback('ModelCloseFcn',gcbh);  PreSaveFcn=simscape.compiler.sli.internal.callback('PreSaveFcn',gcbh);  PostSaveFcn=simscape.compiler.sli.internal.callback('PostSaveFcn',gcbh);  PreCopyFcn=simscape.compiler.sli.internal.callback('PreCopyFcn',gcbh);  PreDeleteFcn=simscape.compiler.sli.internal.callback('PreDeleteFcn',gcbh);
      mask Help: web(nesl_help(gcbh))
      mask TypeOptions P_conf: compiletime | runtime
      mask Display:
      | color('red');
      | port_label('RConn', 1,'');
      | port_label('LConn', 1,'');
